simulink model "gSSVEP_MinimumEnergy"  (Simulink 8.6)
settings: Solver=FixedStepDiscrete  StartTime=0.0  StopTime=260  FixedStep=1/256  RelTol=1e-3
libraries: dspstat3 x2, simulink x1, Tools x1, dspbuff3 x1, gRTanalyze x1, instrumentlib x1
Description:
  | g.USBamp based SSVEP based BCI
  | 
  | Copyright g.tec medical engineering GmbH
settings Model: Creator=g.tec medical engineering GmbH  ModifiedByFormat=g.tec  LastModifiedBy=g.tec
settings DebuggingCC: FcnCallInpInsideContextMsg=UseLocalSettings

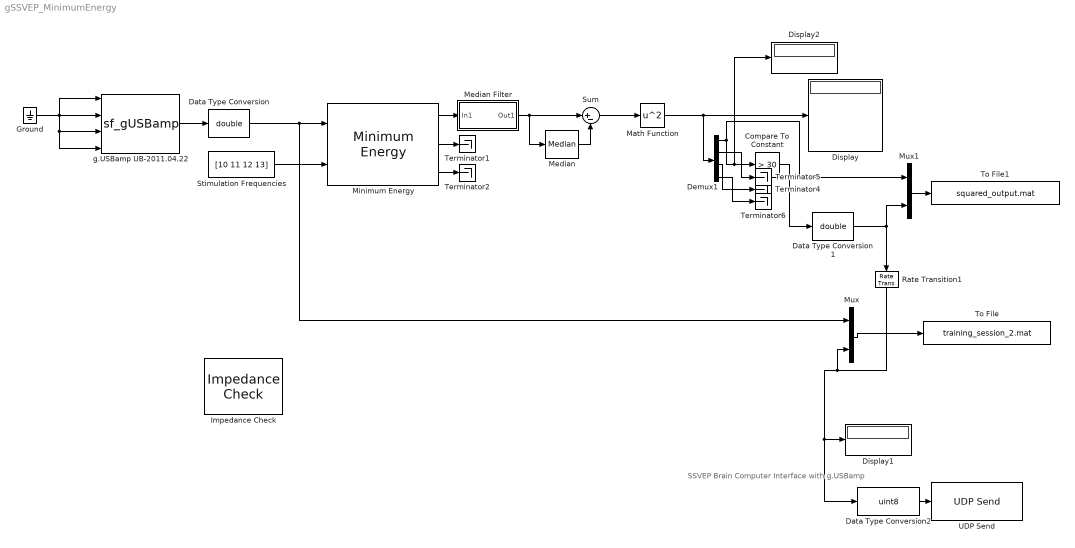
== system gSSVEP_MinimumEnergy ==
  note: SSVEP Brain Computer Interface with g.USBamp
  Compare To Constant : simulink/Logic and Bit Operations/Compare To Constant  relop=>  const=30  OutDataTypeStr=boolean
  Data Type Conversion : DataTypeConversion  OutDataTypeStr=double
  Data Type Conversion1 : DataTypeConversion  OutDataTypeStr=double
  Data Type Conversion2 : DataTypeConversion  OutDataTypeStr=uint8
  Demux1 : Demux
  Display : Display
  Display1 : Display
  Display2 : Display
  Ground : Ground
  Impedance Check : Tools/Impedance Check
  Math Function : Math  Operator=square  SaturateOnIntegerOverflow=on
  Median : dspstat3/Median  sortAlg=Quick sort  directionMode=Entire input  dimension=1  outputDataTypeStr=Inherit: Same as accumulator  outputLastDataTypeStr=Inherit: Same as accumulator  outputMin=[]  outputMax=[]  accumDataTypeStr=Inherit: Same as product output  accumLastDataTypeStr=Inherit: Same as product output  roundingMode=Floor  overflowMode=off
      settings: allowOverrides=off
  Median Filter : Subsystem  mask(Moving Median Filter){buflen=10}
      mask prompts: buflen "Filter Length"
      mask help:
      | Smoothes the input channels over time by computing the median value for
      | the specified number of samples.
      mask init:
      | blockhandle = get_param(gcb,'Handle');
      | sysname = get(blockhandle,'Path');
      | syspath = [ sysname '/' ];
      | name = [ syspath get(blockhandle,'Name') ];
      | path = [ name '/' ];
      | if buflen < 3
      |   buflen = 10;
      |   set_param(name,'buflen',num2str(buflen));
      | end
      | set_param([ path 'Collect'],'siz',num2str(buflen));
      | try
      |   set_param([ path 'Collect'],'TreatMby1Signals','M channels (this choice will be removed - see release notes)');
      | catch
      | end
      mask Help:
      | Smoothes the input channels over time by computing the median value for
      | the specified number of samples.
      | 
      | Filter Length ... The length of the smoothing window in samples. (Default 10)
  Minimum Energy : gRTanalyze/Minimum Energy  bufflen=768  reprate=0.20  numharmonics=1  modelorder=7
  Mux : Mux  Inputs=2
  Mux1 : Mux  Inputs=2
  Rate Transition1 : RateTransition
  Stimulation Frequencies : Constant  Value=[10 11 12 13]  SampleTime=1/256
  Sum : Sum  Inputs=|+-
  Terminator{1..2,4..6} (5 alike) : Terminator
  To File : ToFile  Filename=training_session_2.mat  MatrixName=y
  To File1 : ToFile  Filename=squared_output.mat  MatrixName=y
  UDP Send : instrumentlib/UDP Send  Host=172.22.11.2  Port=1111  LocalPort=-1  EnableBlockingMode=on  ByteOrder=BigEndian
  g.USBamp UB-2011.04.22 : S-Function  FunctionName=sf_gUSBamp  Parameters=cfg,snr  SFunctionDeploymentMode=off  EnableBusSupport=off  mask{cfg=currentCFG_gSSVEP_MinimumEnergy_UB-2011.04.22.cfg, snr=UB-2011.04.22}
      mask prompts: cfg "Configuration"; snr "Serial"
      mask help: Enter configuration file and serial
      settings: OpenFcn=|
      | %gua_click
      | gua_block_cfg
      mask Display: image(imread('USB_symb.tif'))
  wires:
  Stimulation Frequencies/1 -> Minimum Energy/2
  Minimum Energy/1 -> Median Filter/1(In1)
  Median Filter/1(Out1) -> Sum/1, Median/1
  Minimum Energy/2 -> Terminator1/1
  Minimum Energy/3 -> Terminator2/1
  g.USBamp UB-2011.04.22/1 -> Data Type Conversion/1
  Data Type Conversion/1 -> Mux/1, Minimum Energy/1
  Mux/1 -> To File/1
  Rate Transition1/1 -> Mux/2, Data Type Conversion2/1, Display1/1
  Median/1 -> Sum/2
  Ground/1 -> g.USBamp UB-2011.04.22/2, g.USBamp UB-2011.04.22/1, g.USBamp UB-2011.04.22/4, g.USBamp UB-2011.04.22/3
  Sum/1 -> Math Function/1
  Math Function/1 -> Demux1/1, Display/1
  Demux1/1 -> Mux1/1, Display2/1, Compare To Constant/1
  Demux1/2 -> Terminator5/1
  Demux1/3 -> Terminator4/1
  Demux1/4 -> Terminator6/1
  Compare To Constant/1 -> Data Type Conversion1/1
  Data Type Conversion1/1 -> Rate Transition1/1, Mux1/2
  Mux1/1 -> To File1/1
  Data Type Conversion2/1 -> UDP Send/1

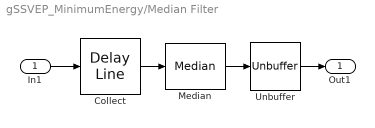
== system gSSVEP_MinimumEnergy/Median Filter ==
  In1 : Inport
  Collect : dspbuff3/Delay Line  siz=10  ic=0  directfeed=on  enable_output=off  hold_output=off  TreatMby1Signals=M channels (this choice will be removed - see release notes)  OutputFrames=on
  Median : dspstat3/Median  sortAlg=Quick sort  directionMode=Specified dimension  dimension=1  outputDataTypeStr=Inherit: Same as accumulator  outputLastDataTypeStr=Inherit: Same as accumulator  outputMin=[]  outputMax=[]  accumDataTypeStr=Inherit: Same as product output  accumLastDataTypeStr=Inherit: Same as product output  roundingMode=Floor  overflowMode=off
      settings: allowOverrides=off
  Unbuffer : Unbuffer
  Out1 : Outport
  wires:
  Unbuffer/1 -> Out1/1
  Median/1 -> Unbuffer/1
  Collect/1 -> Median/1
  In1/1 -> Collect/1
